simulink model "ElevatorPlant_basic"  (R2015b)
(part 3 of 3)

          Emergency.OpCl.OpCl_1.Closing1.Flag_floor -> (junction 23694)
          (junction 23694) -> (junction 23693)
          (junction 23693) -> (junction 23696)
          Emergency.OpCl.OpCl_1.Closing1.Stop_Closing1 -> (junction 23695)
          (junction 23695) -> (junction 23696)
        state StopClosing
          en: CP1=false;
          FLAG_OD=false;
        state Opening1
          state Opening
            en:AP1=Q_op;
          state Stop_Opening
            en:AP1=false;
            FLAG_OD=true;
            OBS=true;
            IN_op=false;
            ET_op=0;
          state Timer_open
            state Set_tmr
              en: Q_op=true;
            state Set
              en:PT_op=2;
              IN_op=true;
            state Counting
              en:ET_op = ET_op + 1;
              Q_op=false;
            (junction 23815) -> Emergency.OpCl.OpCl_1.Opening1.Timer_open.Set_tmr [order 1] : [ET_op==PT_op]
            Emergency.OpCl.OpCl_1.Opening1.Timer_open.Set_tmr -> (junction 23816)
            (default) -> Emergency.OpCl.OpCl_1.Opening1.Timer_open.Set
            Emergency.OpCl.OpCl_1.Opening1.Timer_open.Counting -> (junction 23815)
            (junction 23815) -> (junction 23816) [order 2]
            Emergency.OpCl.OpCl_1.Opening1.Timer_open.Set -> (junction 23817)
            (junction 23817) -> Emergency.OpCl.OpCl_1.Opening1.Timer_open.Counting [order 1] : [ET_op<PT_op]
            (junction 23817) -> (junction 23816) [order 2]
          state BUTT_Temp
            state Butt_temp0
              en: BUT_TEMP = 0;
              FLAG_BT=true;
              LPC0=true;
            state Butt_temp1
              en: BUT_TEMP = 1;
              FLAG_BT=true;
              LPC1=true;
            state Butt_temp2
              en: BUT_TEMP = 2;
              FLAG_BT=true;
              LPC2=true;
            state Butt_temp3
              en: BUT_TEMP = 3;
              FLAG_BT=true;
              LPC3=true;
            (default) -> (junction 23830)
            (junction 23830) -> (junction 23831) [order 1] : [not(FLAG_BT)]
            (junction 23831) -> Emergency.OpCl.OpCl_1.Opening1.BUTT_Temp.Butt_temp0 [order 1] : [P0]
            Emergency.OpCl.OpCl_1.Opening1.BUTT_Temp.Butt_temp0 -> (junction 23832)
            (junction 23831) -> (junction 23834) [order 2]
            (junction 23832) -> (junction 23833)
            (junction 23830) -> (junction 23841) [order 2]
            Emergency.OpCl.OpCl_1.Opening1.BUTT_Temp.Butt_temp1 -> (junction 23833)
            (junction 23834) -> Emergency.OpCl.OpCl_1.Opening1.BUTT_Temp.Butt_temp1 [order 1] : [P1]
            (junction 23833) -> (junction 23836)
            (junction 23834) -> (junction 23835) [order 2]
            (junction 23835) -> Emergency.OpCl.OpCl_1.Opening1.BUTT_Temp.Butt_temp2 [order 1] : [P2]
            Emergency.OpCl.OpCl_1.Opening1.BUTT_Temp.Butt_temp2 -> (junction 23836)
            (junction 23835) -> (junction 23837) [order 2]
            (junction 23836) -> (junction 23838)
            (junction 23837) -> Emergency.OpCl.OpCl_1.Opening1.BUTT_Temp.Butt_temp3 [order 1] : [P3]
            Emergency.OpCl.OpCl_1.Opening1.BUTT_Temp.Butt_temp3 -> (junction 23838)
            (junction 23838) -> (junction 23840)
            (junction 23837) -> (junction 23839) [order 2]
            (junction 23840) -> (junction 23839)
            (junction 23839) -> (junction 23842)
            (junction 23841) -> (junction 23842)
          state BUTT_Temp1
            state Butt_temp0
              en: BUT_TEMP = 0;
              FLAG_BT=true;
              LPC0=true;
            state Butt_temp1
              en: BUT_TEMP = 1;
              FLAG_BT=true;
              LPC1=true;
            state Butt_temp2
              en: BUT_TEMP = 2;
              FLAG_BT=true;
              LPC2=true;
            state Butt_temp3
              en: BUT_TEMP = 3;
              FLAG_BT=true;
              LPC3=true;
            (default) -> (junction 23870)
            (junction 23870) -> (junction 23871) [order 1] : [not(FLAG_BT)]
            (junction 23871) -> Emergency.OpCl.OpCl_1.Opening1.BUTT_Temp1.Butt_temp0 [order 1] : [P0]
            Emergency.OpCl.OpCl_1.Opening1.BUTT_Temp1.Butt_temp0 -> (junction 23872)
            (junction 23871) -> (junction 23874) [order 2]
            (junction 23872) -> (junction 23873)
            (junction 23870) -> (junction 23881) [order 2]
            Emergency.OpCl.OpCl_1.Opening1.BUTT_Temp1.Butt_temp1 -> (junction 23873)
            (junction 23874) -> Emergency.OpCl.OpCl_1.Opening1.BUTT_Temp1.Butt_temp1 [order 1] : [P1]
            (junction 23873) -> (junction 23876)
            (junction 23874) -> (junction 23875) [order 2]
            (junction 23875) -> Emergency.OpCl.OpCl_1.Opening1.BUTT_Temp1.Butt_temp2 [order 1] : [P2]
            Emergency.OpCl.OpCl_1.Opening1.BUTT_Temp1.Butt_temp2 -> (junction 23876)
            (junction 23875) -> (junction 23877) [order 2]
            (junction 23876) -> (junction 23878)
            (junction 23877) -> Emergency.OpCl.OpCl_1.Opening1.BUTT_Temp1.Butt_temp3 [order 1] : [P3]
            Emergency.OpCl.OpCl_1.Opening1.BUTT_Temp1.Butt_temp3 -> (junction 23878)
            (junction 23878) -> (junction 23880)
            (junction 23877) -> (junction 23879) [order 2]
            (junction 23880) -> (junction 23879)
            (junction 23879) -> (junction 23882)
            (junction 23881) -> (junction 23882)
          state Opening1
            en:AP1=true;
          state People_IN
            state Check_People_IN
              en:
              COUNTER_IN=false;
            state Ready_IN
              en:
              IN_DEL_IN=false;
              ET_DEL_IN=0;
            state People_KID_IN
              en:
              WEIGHT=WEIGHT+30;
              KIDS=KIDS+1;
            state DELAY_IN
              state Set_tmr
                en:
                Q_DEL_IN=true;
              state Counting
                en:
                ET_DEL_IN = ET_DEL_IN + 1;
                Q_DEL_IN=false;
              state Set
                en:
                IN_DEL_IN=true;
                PT_DEL_IN=0.05;
              (junction 23966) -> Emergency.OpCl.OpCl_1.Opening1.People_IN.DELAY_IN.Set_tmr [order 1] : [ET_DEL_IN==PT_DEL_IN]
              Emergency.OpCl.OpCl_1.Opening1.People_IN.DELAY_IN.Set_tmr -> (junction 23967)
              Emergency.OpCl.OpCl_1.Opening1.People_IN.DELAY_IN.Counting -> (junction 23966)
              (junction 23966) -> (junction 23967) [order 2]
              (default) -> Emergency.OpCl.OpCl_1.Opening1.People_IN.DELAY_IN.Set
              Emergency.OpCl.OpCl_1.Opening1.People_IN.DELAY_IN.Set -> (junction 23968)
              (junction 23968) -> Emergency.OpCl.OpCl_1.Opening1.People_IN.DELAY_IN.Counting [order 1] : [ET_DEL_IN<PT_DEL_IN]
              (junction 23968) -> (junction 23967) [order 2]
            state People_WOMAN_IN
              en:
              WEIGHT=WEIGHT+55;
              WOMEN=WOMEN+1;
            state People_MAN_IN
              en:
              WEIGHT=WEIGHT+75;
              MEN=MEN+1;
            state People_FATGUY_IN
              en:
              WEIGHT=WEIGHT+100;
              FATGUYS=FATGUYS+1;
            state Re_Ready_IN
              en:
              COUNTER_IN=true;
            Emergency.OpCl.OpCl_1.Opening1.People_IN.Check_People_IN -> (junction 23911)
            (junction 23911) -> Emergency.OpCl.OpCl_1.Opening1.People_IN.People_KID_IN [order 1] : [KID_IN]
            Emergency.OpCl.OpCl_1.Opening1.People_IN.People_KID_IN -> (junction 23912)
            Emergency.OpCl.OpCl_1.Opening1.People_IN.DELAY_IN -> (junction 23913)
            (junction 23913) -> Emergency.OpCl.OpCl_1.Opening1.People_IN.Ready_IN [order 1] : [Q_DEL_IN]
            (default) -> Emergency.OpCl.OpCl_1.Opening1.People_IN.DELAY_IN
            Emergency.OpCl.OpCl_1.Opening1.People_IN.Ready_IN -> (junction 23914)
            (junction 23914) -> Emergency.OpCl.OpCl_1.Opening1.People_IN.Check_People_IN [order 1] : [COUNTER_IN]
            (junction 23911) -> (junction 23916) [order 2]
            (junction 23912) -> (junction 23915)
            (junction 23913) -> (junction 23925) [order 2]
            (junction 23914) -> (junction 23924) [order 2]
            (junction 23916) -> Emergency.OpCl.OpCl_1.Opening1.People_IN.People_WOMAN_IN [order 1] : [WOMAN_IN]
            Emergency.OpCl.OpCl_1.Opening1.People_IN.People_WOMAN_IN -> (junction 23915)
            (junction 23916) -> (junction 23917) [order 2]
            (junction 23915) -> (junction 23918)
            (junction 23917) -> Emergency.OpCl.OpCl_1.Opening1.People_IN.People_MAN_IN [order 1] : [MAN_IN]
            Emergency.OpCl.OpCl_1.Opening1.People_IN.People_MAN_IN -> (junction 23918)
            (junction 23917) -> (junction 23919) [order 2]
            (junction 23918) -> (junction 23920)
            (junction 23919) -> Emergency.OpCl.OpCl_1.Opening1.People_IN.People_FATGUY_IN [order 1] : [FATGUY_IN]
            Emergency.OpCl.OpCl_1.Opening1.People_IN.People_FATGUY_IN -> (junction 23920)
            (junction 23919) -> (junction 23921) [order 2]
            (junction 23920) -> (junction 23922)
            (junction 23921) -> (junction 23922)
            (junction 23922) -> (junction 23923)
            (junction 23924) -> (junction 23923)
            (junction 23923) -> (junction 23926)
            (junction 23925) -> (junction 23926)
            (junction 23926) -> (junction 23927)
            (junction 23927) -> Emergency.OpCl.OpCl_1.Opening1.People_IN.Re_Ready_IN [order 1] : [not(KID_IN|| WOMAN_IN || MAN_IN || FATGUY_IN)]
            (junction 23927) -> (junction 23928) [order 2]
            Emergency.OpCl.OpCl_1.Opening1.People_IN.Re_Ready_IN -> (junction 23928)
          state People_OUT
            state Ready_OUT
              en:
              IN_DEL_OUT=false;
              ET_DEL_OUT=0;
            state Check_People_OUT
              en:
              COUNTER_OUT=false;
            state People_KID_OUT
              en:
              WEIGHT=WEIGHT-30;
              KIDS=KIDS-1;
            state DELAY_OUT
              state Set_tmr
                en:
                Q_DEL_OUT=true;
              state Counting
                en:
                ET_DEL_OUT = ET_DEL_OUT + 1;
                Q_DEL_OUT=false;
              state Set
                en:
                IN_DEL_OUT=true;
                PT_DEL_OUT=0.05;
              (junction 24040) -> Emergency.OpCl.OpCl_1.Opening1.People_OUT.DELAY_OUT.Set_tmr [order 1] : [ET_DEL_OUT==PT_DEL_OUT]
              Emergency.OpCl.OpCl_1.Opening1.People_OUT.DELAY_OUT.Set_tmr -> (junction 24041)
              Emergency.OpCl.OpCl_1.Opening1.People_OUT.DELAY_OUT.Counting -> (junction 24040)
              (junction 24040) -> (junction 24041) [order 2]
              (default) -> Emergency.OpCl.OpCl_1.Opening1.People_OUT.DELAY_OUT.Set
              Emergency.OpCl.OpCl_1.Opening1.People_OUT.DELAY_OUT.Set -> (junction 24042)
              (junction 24042) -> Emergency.OpCl.OpCl_1.Opening1.People_OUT.DELAY_OUT.Counting [order 1] : [ET_DEL_OUT<PT_DEL_OUT]
              (junction 24042) -> (junction 24041) [order 2]
            state People_WOMAN_OUT
              en:
              WEIGHT=WEIGHT-55;
              WOMEN=WOMEN-1;
            state People_MAN_OUT
              en:
              WEIGHT=WEIGHT-75;
              MEN=MEN-1;
            state People_FATGUY_OUT
              en:
              WEIGHT=WEIGHT-100;
              FATGUYS=FATGUYS-1;
            state Re_Ready_OUT
              en:
              COUNTER_OUT=true;
            (default) -> Emergency.OpCl.OpCl_1.Opening1.People_OUT.DELAY_OUT
            Emergency.OpCl.OpCl_1.Opening1.People_OUT.DELAY_OUT -> (junction 23985)
            (junction 23985) -> Emergency.OpCl.OpCl_1.Opening1.People_OUT.Ready_OUT [order 1] : [Q_DEL_OUT]
            Emergency.OpCl.OpCl_1.Opening1.People_OUT.Ready_OUT -> (junction 23986)
            (junction 23986) -> Emergency.OpCl.OpCl_1.Opening1.People_OUT.Check_People_OUT [order 1] : [COUNTER_OUT]
            Emergency.OpCl.OpCl_1.Opening1.People_OUT.Check_People_OUT -> (junction 23987)
            (junction 23987) -> Emergency.OpCl.OpCl_1.Opening1.People_OUT.People_KID_OUT [order 1] : [KID_OUT && KIDS>0 ]
            Emergency.OpCl.OpCl_1.Opening1.People_OUT.People_KID_OUT -> (junction 23988)
            (junction 23985) -> (junction 23999) [order 2]
            (junction 23986) -> (junction 23997) [order 2]
            (junction 23987) -> (junction 23989) [order 2]
            (junction 23988) -> (junction 23990)
            (junction 23989) -> Emergency.OpCl.OpCl_1.Opening1.People_OUT.People_WOMAN_OUT [order 1] : [WOMAN_OUT && WOMEN>0]
            Emergency.OpCl.OpCl_1.Opening1.People_OUT.People_WOMAN_OUT -> (junction 23990)
            (junction 23989) -> (junction 23992) [order 2]
            (junction 23990) -> (junction 23991)
            (junction 23992) -> Emergency.OpCl.OpCl_1.Opening1.People_OUT.People_MAN_OUT [order 1] : [MAN_OUT && MEN>0]
            Emergency.OpCl.OpCl_1.Opening1.People_OUT.People_MAN_OUT -> (junction 23991)
            (junction 23992) -> (junction 23993) [order 2]
            (junction 23991) -> (junction 23994)
            (junction 23993) -> Emergency.OpCl.OpCl_1.Opening1.People_OUT.People_FATGUY_OUT [order 1] : [FATGUY_OUT && FATGUYS>0]
            Emergency.OpCl.OpCl_1.Opening1.People_OUT.People_FATGUY_OUT -> (junction 23994)
            (junction 23993) -> (junction 23996) [order 2]
            (junction 23994) -> (junction 23995)
            (junction 23996) -> (junction 23995)
            (junction 23995) -> (junction 23998)
            (junction 23997) -> (junction 23998)
            (junction 23998) -> (junction 24000)
            (junction 23999) -> (junction 24000)
            (junction 24000) -> (junction 24001)
            (junction 24001) -> Emergency.OpCl.OpCl_1.Opening1.People_OUT.Re_Ready_OUT [order 1] : [not(KID_OUT || WOMAN_OUT || MAN_OUT || FATGUY_OUT)]
            (junction 24001) -> (junction 24002) [order 2]
            Emergency.OpCl.OpCl_1.Opening1.People_OUT.Re_Ready_OUT -> (junction 24002)
          state Stop_Opening1
            en: AP1=false;
            FLAG_OD=true;
            IN_cl=false;
            ET_cl=0;
          Emergency.OpCl.OpCl_1.Opening1.Opening -> (junction 23781)
          (junction 23781) -> (junction 23780)
          Emergency.OpCl.OpCl_1.Opening1.Stop_Opening -> (junction 23781)
          (junction 23780) -> (junction 23784)
          (junction 23783) -> Emergency.OpCl.OpCl_1.Opening1.Opening [order 1] : [not(PA1)]
          (junction 23782) -> Emergency.OpCl.OpCl_1.Opening1.BUTT_Temp [order 1] : [not(FLAG==4)]
          Emergency.OpCl.OpCl_1.Opening1.BUTT_Temp -> (junction 23783)
          (junction 23783) -> Emergency.OpCl.OpCl_1.Opening1.Stop_Opening [order 2]
          Emergency.OpCl.OpCl_1.Opening1.Timer_open -> (junction 23782)
          (junction 23782) -> (junction 23783) [order 2]
          (junction 23786) -> Emergency.OpCl.OpCl_1.Opening1.Timer_open [order 1] : [not(OBS)]
          Emergency.OpCl.OpCl_1.Opening1.Opening1 -> (junction 23784)
          (junction 23785) -> Emergency.OpCl.OpCl_1.Opening1.Opening1 [order 1] : [not(PA1)]
          Emergency.OpCl.OpCl_1.Opening1.BUTT_Temp1 -> (junction 23785)
          Emergency.OpCl.OpCl_1.Opening1.People_IN -> Emergency.OpCl.OpCl_1.Opening1.People_OUT
          Emergency.OpCl.OpCl_1.Opening1.People_OUT -> (junction 23786)
          (junction 23786) -> (junction 23787) [order 2]
          (junction 23787) -> Emergency.OpCl.OpCl_1.Opening1.BUTT_Temp1 [order 1] : [not(FLAG==4)]
          (default) -> Emergency.OpCl.OpCl_1.Opening1.People_IN
          (junction 23787) -> (junction 23785) [order 2]
          (junction 23788) -> (junction 23784)
          (junction 23785) -> Emergency.OpCl.OpCl_1.Opening1.Stop_Opening1 [order 2]
          Emergency.OpCl.OpCl_1.Opening1.Stop_Opening1 -> (junction 23788)
        (default) -> (junction 23673)
        (junction 23673) -> (junction 23674) [order 1] : [FLAG_OD]
        (junction 23674) -> Emergency.OpCl.OpCl_1.Closing1 [order 1] : [not(SWITCH) && not(STOP) && WEIGHT<=320 && not(PS1 || PD1 || P1) ]
        (junction 23673) -> Emergency.OpCl.OpCl_1.Opening1 [order 2]
        (junction 23674) -> Emergency.OpCl.OpCl_1.StopClosing [order 2]
        Emergency.OpCl.OpCl_1.Closing1 -> (junction 23675)
        Emergency.OpCl.OpCl_1.StopClosing -> (junction 23675)
        (junction 23675) -> (junction 23676)
        Emergency.OpCl.OpCl_1.Opening1 -> (junction 23676)
      state FLOOR_2
        en: CP2=false;
      state OpCl_2
        state Closing2
          state Timer_close
            state Set_tmr
              en: Q_cl=true;
            state Set
              en:PT_cl=5;
              IN_cl=true;
            state Counting
              en:ET_cl = ET_cl + 1;
              Q_cl=false;
            (junction 24494) -> Emergency.OpCl.OpCl_2.Closing2.Timer_close.Set_tmr [order 1] : [ET_cl==PT_cl]
            Emergency.OpCl.OpCl_2.Closing2.Timer_close.Set_tmr -> (junction 24495)
            (default) -> Emergency.OpCl.OpCl_2.Closing2.Timer_close.Set
            Emergency.OpCl.OpCl_2.Closing2.Timer_close.Counting -> (junction 24494)
            (junction 24494) -> (junction 24495) [order 2]
            Emergency.OpCl.OpCl_2.Closing2.Timer_close.Set -> (junction 24496)
            (junction 24496) -> Emergency.OpCl.OpCl_2.Closing2.Timer_close.Counting [order 1] : [ET_cl<PT_cl]
            (junction 24496) -> (junction 24495) [order 2]
          state BUTT_Temp
            state Butt_temp0
              en: BUT_TEMP = 0;
              FLAG_BT=true;
              LPC0=true;
            state Butt_temp1
              en: BUT_TEMP = 1;
              FLAG_BT=true;
              LPC1=true;
            state Butt_temp2
              en: BUT_TEMP = 2;
              FLAG_BT=true;
              LPC2=true;
            state Butt_temp3
              en: BUT_TEMP = 3;
              FLAG_BT=true;
              LPC3=true;
            (default) -> (junction 24509)
            (junction 24509) -> (junction 24510) [order 1] : [not(FLAG_BT)]
            (junction 24510) -> Emergency.OpCl.OpCl_2.Closing2.BUTT_Temp.Butt_temp0 [order 1] : [P0]
            Emergency.OpCl.OpCl_2.Closing2.BUTT_Temp.Butt_temp0 -> (junction 24511)
            (junction 24509) -> (junction 24518) [order 2]
            (junction 24510) -> (junction 24513) [order 2]
            (junction 24511) -> (junction 24512)
            (junction 24513) -> Emergency.OpCl.OpCl_2.Closing2.BUTT_Temp.Butt_temp1 [order 1] : [P1]
            Emergency.OpCl.OpCl_2.Closing2.BUTT_Temp.Butt_temp1 -> (junction 24512)
            (junction 24513) -> (junction 24514) [order 2]
            (junction 24512) -> (junction 24515)
            (junction 24514) -> Emergency.OpCl.OpCl_2.Closing2.BUTT_Temp.Butt_temp2 [order 1] : [P2]
            Emergency.OpCl.OpCl_2.Closing2.BUTT_Temp.Butt_temp2 -> (junction 24515)
            (junction 24514) -> (junction 24516) [order 2]
            (junction 24515) -> (junction 24517)
            (junction 24516) -> Emergency.OpCl.OpCl_2.Closing2.BUTT_Temp.Butt_temp3 [order 1] : [P3]
            Emergency.OpCl.OpCl_2.Closing2.BUTT_Temp.Butt_temp3 -> (junction 24517)
            (junction 24516) -> (junction 24519) [order 2]
            (junction 24517) -> (junction 24520)
            (junction 24518) -> (junction 24519)
            (junction 24519) -> (junction 24520)
          state Closing
            en: CP2=Q_cl;
          state Stop_Closing
            en: CP2=false;
            LPS0=false;
            LPS1=false;
            LPD1=false;
            LPS2=false;
            LPD2=false;
            LPD3=false;
            FLAG_OD=false;
            OBS=false;
            ET_cl=0;
            IN_cl=false;
          state Flag_position
            en:FLAG=2;
            FLAG_BT=false;
            BUTTON=BUT_TEMP;
          state Closing1
            en:CP2=true;
          state Flag_floor
            en: FLAG=1;
          state Stop_Closing1
            en:CP2=false;
          Emergency.OpCl.OpCl_2.Closing2.Closing -> Emergency.OpCl.OpCl_2.Closing2.BUTT_Temp
          (default) -> (junction 24461)
          (junction 24461) -> Emergency.OpCl.OpCl_2.Closing2.Timer_close [order 1] : [not(FLAG==0) && not(FLAG==4)]
          Emergency.OpCl.OpCl_2.Closing2.Timer_close -> (junction 24462)
          Emergency.OpCl.OpCl_2.Closing2.BUTT_Temp -> (junction 24463)
          (junction 24462) -> Emergency.OpCl.OpCl_2.Closing2.Closing [order 1] : [not(PC2)]
          (junction 24461) -> (junction 24465) [order 2]
          (junction 24462) -> Emergency.OpCl.OpCl_2.Closing2.Stop_Closing [order 2]
          (junction 24463) -> (junction 24467)
          Emergency.OpCl.OpCl_2.Closing2.Stop_Closing -> (junction 24464)
          (junction 24464) -> Emergency.OpCl.OpCl_2.Closing2.Flag_position [order 1] : [FLAG_BT]
          (junction 24464) -> Emergency.OpCl.OpCl_2.Closing2.Flag_floor [order 2]
          Emergency.OpCl.OpCl_2.Closing2.Flag_position -> (junction 24468)
          (junction 24465) -> Emergency.OpCl.OpCl_2.Closing2.Closing1 [order 1] : [not(PC2)]
          Emergency.OpCl.OpCl_2.Closing2.Closing1 -> (junction 24466)
          (junction 24465) -> Emergency.OpCl.OpCl_2.Closing2.Stop_Closing1 [order 2]
          (junction 24466) -> (junction 24469)
          Emergency.OpCl.OpCl_2.Closing2.Flag_floor -> (junction 24468)
          (junction 24468) -> (junction 24467)
          (junction 24467) -> (junction 24470)
          Emergency.OpCl.OpCl_2.Closing2.Stop_Closing1 -> (junction 24469)
          (junction 24469) -> (junction 24470)
        state StopClosing
          en: CP2=false;
          FLAG_OD=false;
        state Opening2
          state Opening
            en:AP2=Q_op;
          state Stop_Opening
            en:AP2=false;
            FLAG_OD=true;
            OBS=true;
            IN_op=false;
            ET_op=0;
          state Timer_open
            state Set_tmr
              en: Q_op=true;
            state Set
              en:PT_op=2;
              IN_op=true;
            state Counting
              en:ET_op = ET_op + 1;
              Q_op=false;
            (junction 24589) -> Emergency.OpCl.OpCl_2.Opening2.Timer_open.Set_tmr [order 1] : [ET_op==PT_op]
            Emergency.OpCl.OpCl_2.Opening2.Timer_open.Set_tmr -> (junction 24590)
            (default) -> Emergency.OpCl.OpCl_2.Opening2.Timer_open.Set
            Emergency.OpCl.OpCl_2.Opening2.Timer_open.Counting -> (junction 24589)
            (junction 24589) -> (junction 24590) [order 2]
            Emergency.OpCl.OpCl_2.Opening2.Timer_open.Set -> (junction 24591)
            (junction 24591) -> Emergency.OpCl.OpCl_2.Opening2.Timer_open.Counting [order 1] : [ET_op<PT_op]
            (junction 24591) -> (junction 24590) [order 2]
          state BUTT_Temp
            state Butt_temp0
              en: BUT_TEMP = 0;
              FLAG_BT=true;
              LPC0=true;
            state Butt_temp1
              en: BUT_TEMP = 1;
              FLAG_BT=true;
              LPC1=true;
            state Butt_temp2
              en: BUT_TEMP = 2;
              FLAG_BT=true;
              LPC2=true;
            state Butt_temp3
              en: BUT_TEMP = 3;
              FLAG_BT=true;
              LPC3=true;
            (default) -> (junction 24604)
            (junction 24604) -> (junction 24605) [order 1] : [not(FLAG_BT)]
            (junction 24605) -> Emergency.OpCl.OpCl_2.Opening2.BUTT_Temp.Butt_temp0 [order 1] : [P0]
            Emergency.OpCl.OpCl_2.Opening2.BUTT_Temp.Butt_temp0 -> (junction 24606)
            (junction 24605) -> (junction 24608) [order 2]
            (junction 24606) -> (junction 24607)
            (junction 24604) -> (junction 24615) [order 2]
            Emergency.OpCl.OpCl_2.Opening2.BUTT_Temp.Butt_temp1 -> (junction 24607)
            (junction 24608) -> Emergency.OpCl.OpCl_2.Opening2.BUTT_Temp.Butt_temp1 [order 1] : [P1]
            (junction 24607) -> (junction 24610)
            (junction 24608) -> (junction 24609) [order 2]
            (junction 24609) -> Emergency.OpCl.OpCl_2.Opening2.BUTT_Temp.Butt_temp2 [order 1] : [P2]
            Emergency.OpCl.OpCl_2.Opening2.BUTT_Temp.Butt_temp2 -> (junction 24610)
            (junction 24609) -> (junction 24611) [order 2]
            (junction 24610) -> (junction 24612)
            (junction 24611) -> Emergency.OpCl.OpCl_2.Opening2.BUTT_Temp.Butt_temp3 [order 1] : [P3]
            Emergency.OpCl.OpCl_2.Opening2.BUTT_Temp.Butt_temp3 -> (junction 24612)
            (junction 24612) -> (junction 24614)
            (junction 24611) -> (junction 24613) [order 2]
            (junction 24614) -> (junction 24613)
            (junction 24613) -> (junction 24616)
            (junction 24615) -> (junction 24616)
          state BUTT_Temp1
            state Butt_temp0
              en: BUT_TEMP = 0;
              FLAG_BT=true;
              LPC0=true;
            state Butt_temp1
              en: BUT_TEMP = 1;
              FLAG_BT=true;
              LPC1=true;
            state Butt_temp2
              en: BUT_TEMP = 2;
              FLAG_BT=true;
              LPC2=true;
            state Butt_temp3
              en: BUT_TEMP = 3;
              FLAG_BT=true;
              LPC3=true;
            (default) -> (junction 24644)
            (junction 24644) -> (junction 24645) [order 1] : [not(FLAG_BT)]
            (junction 24645) -> Emergency.OpCl.OpCl_2.Opening2.BUTT_Temp1.Butt_temp0 [order 1] : [P0]
            Emergency.OpCl.OpCl_2.Opening2.BUTT_Temp1.Butt_temp0 -> (junction 24646)
            (junction 24645) -> (junction 24648) [order 2]
            (junction 24646) -> (junction 24647)
            (junction 24644) -> (junction 24655) [order 2]
            Emergency.OpCl.OpCl_2.Opening2.BUTT_Temp1.Butt_temp1 -> (junction 24647)
            (junction 24648) -> Emergency.OpCl.OpCl_2.Opening2.BUTT_Temp1.Butt_temp1 [order 1] : [P1]
            (junction 24647) -> (junction 24650)
            (junction 24648) -> (junction 24649) [order 2]
            (junction 24649) -> Emergency.OpCl.OpCl_2.Opening2.BUTT_Temp1.Butt_temp2 [order 1] : [P2]
            Emergency.OpCl.OpCl_2.Opening2.BUTT_Temp1.Butt_temp2 -> (junction 24650)
            (junction 24649) -> (junction 24651) [order 2]
            (junction 24650) -> (junction 24652)
            (junction 24651) -> Emergency.OpCl.OpCl_2.Opening2.BUTT_Temp1.Butt_temp3 [order 1] : [P3]
            Emergency.OpCl.OpCl_2.Opening2.BUTT_Temp1.Butt_temp3 -> (junction 24652)
            (junction 24652) -> (junction 24654)
            (junction 24651) -> (junction 24653) [order 2]
            (junction 24654) -> (junction 24653)
            (junction 24653) -> (junction 24656)
            (junction 24655) -> (junction 24656)
          state Opening1
            en:AP2=true;
          state People_IN
            state Check_People_IN
              en:
              COUNTER_IN=false;
            state Ready_IN
              en:
              IN_DEL_IN=false;
              ET_DEL_IN=0;
            state People_KID_IN
              en:
              WEIGHT=WEIGHT+30;
              KIDS=KIDS+1;
            state DELAY_IN
              state Set_tmr
                en:
                Q_DEL_IN=true;
              state Counting
                en:
                ET_DEL_IN = ET_DEL_IN + 1;
                Q_DEL_IN=false;
              state Set
                en:
                IN_DEL_IN=true;
                PT_DEL_IN=0.05;
              (junction 24740) -> Emergency.OpCl.OpCl_2.Opening2.People_IN.DELAY_IN.Set_tmr [order 1] : [ET_DEL_IN==PT_DEL_IN]
              Emergency.OpCl.OpCl_2.Opening2.People_IN.DELAY_IN.Set_tmr -> (junction 24741)
              Emergency.OpCl.OpCl_2.Opening2.People_IN.DELAY_IN.Counting -> (junction 24740)
              (junction 24740) -> (junction 24741) [order 2]
              (default) -> Emergency.OpCl.OpCl_2.Opening2.People_IN.DELAY_IN.Set
              Emergency.OpCl.OpCl_2.Opening2.People_IN.DELAY_IN.Set -> (junction 24742)
              (junction 24742) -> Emergency.OpCl.OpCl_2.Opening2.People_IN.DELAY_IN.Counting [order 1] : [ET_DEL_IN<PT_DEL_IN]
              (junction 24742) -> (junction 24741) [order 2]
            state People_WOMAN_IN
              en:
              WEIGHT=WEIGHT+55;
              WOMEN=WOMEN+1;
            state People_MAN_IN
              en:
              WEIGHT=WEIGHT+75;
              MEN=MEN+1;
            state People_FATGUY_IN
              en:
              WEIGHT=WEIGHT+100;
              FATGUYS=FATGUYS+1;
            state Re_Ready_IN
              en:
              COUNTER_IN=true;
            Emergency.OpCl.OpCl_2.Opening2.People_IN.Check_People_IN -> (junction 24685)
            (junction 24685) -> Emergency.OpCl.OpCl_2.Opening2.People_IN.People_KID_IN [order 1] : [KID_IN]
            Emergency.OpCl.OpCl_2.Opening2.People_IN.People_KID_IN -> (junction 24686)
            Emergency.OpCl.OpCl_2.Opening2.People_IN.DELAY_IN -> (junction 24687)
            (junction 24687) -> Emergency.OpCl.OpCl_2.Opening2.People_IN.Ready_IN [order 1] : [Q_DEL_IN]
            (default) -> Emergency.OpCl.OpCl_2.Opening2.People_IN.DELAY_IN
            Emergency.OpCl.OpCl_2.Opening2.People_IN.Ready_IN -> (junction 24688)
            (junction 24688) -> Emergency.OpCl.OpCl_2.Opening2.People_IN.Check_People_IN [order 1] : [COUNTER_IN]
            (junction 24685) -> (junction 24690) [order 2]
            (junction 24686) -> (junction 24689)
            (junction 24687) -> (junction 24699) [order 2]
            (junction 24688) -> (junction 24698) [order 2]
            (junction 24690) -> Emergency.OpCl.OpCl_2.Opening2.People_IN.People_WOMAN_IN [order 1] : [WOMAN_IN]
            Emergency.OpCl.OpCl_2.Opening2.People_IN.People_WOMAN_IN -> (junction 24689)
            (junction 24690) -> (junction 24691) [order 2]
            (junction 24689) -> (junction 24692)
            (junction 24691) -> Emergency.OpCl.OpCl_2.Opening2.People_IN.People_MAN_IN [order 1] : [MAN_IN]
            Emergency.OpCl.OpCl_2.Opening2.People_IN.People_MAN_IN -> (junction 24692)
            (junction 24691) -> (junction 24693) [order 2]
            (junction 24692) -> (junction 24694)
            (junction 24693) -> Emergency.OpCl.OpCl_2.Opening2.People_IN.People_FATGUY_IN [order 1] : [FATGUY_IN]
            Emergency.OpCl.OpCl_2.Opening2.People_IN.People_FATGUY_IN -> (junction 24694)
            (junction 24693) -> (junction 24695) [order 2]
            (junction 24694) -> (junction 24696)
            (junction 24695) -> (junction 24696)
            (junction 24696) -> (junction 24697)
            (junction 24698) -> (junction 24697)
            (junction 24697) -> (junction 24700)
            (junction 24699) -> (junction 24700)
            (junction 24700) -> (junction 24701)
            (junction 24701) -> Emergency.OpCl.OpCl_2.Opening2.People_IN.Re_Ready_IN [order 1] : [not(KID_IN|| WOMAN_IN || MAN_IN || FATGUY_IN)]
            (junction 24701) -> (junction 24702) [order 2]
            Emergency.OpCl.OpCl_2.Opening2.People_IN.Re_Ready_IN -> (junction 24702)
          state People_OUT
            state Ready_OUT
              en:
              IN_DEL_OUT=false;
              ET_DEL_OUT=0;
            state Check_People_OUT
              en:
              COUNTER_OUT=false;
            state People_KID_OUT
              en:
              WEIGHT=WEIGHT-30;
              KIDS=KIDS-1;
            state DELAY_OUT
              state Set_tmr
                en:
                Q_DEL_OUT=true;
              state Counting
                en:
                ET_DEL_OUT = ET_DEL_OUT + 1;
                Q_DEL_OUT=false;
              state Set
                en:
                IN_DEL_OUT=true;
                PT_DEL_OUT=0.05;
              (junction 24814) -> Emergency.OpCl.OpCl_2.Opening2.People_OUT.DELAY_OUT.Set_tmr [order 1] : [ET_DEL_OUT==PT_DEL_OUT]
              Emergency.OpCl.OpCl_2.Opening2.People_OUT.DELAY_OUT.Set_tmr -> (junction 24815)
              Emergency.OpCl.OpCl_2.Opening2.People_OUT.DELAY_OUT.Counting -> (junction 24814)
              (junction 24814) -> (junction 24815) [order 2]
              (default) -> Emergency.OpCl.OpCl_2.Opening2.People_OUT.DELAY_OUT.Set
              Emergency.OpCl.OpCl_2.Opening2.People_OUT.DELAY_OUT.Set -> (junction 24816)
              (junction 24816) -> Emergency.OpCl.OpCl_2.Opening2.People_OUT.DELAY_OUT.Counting [order 1] : [ET_DEL_OUT<PT_DEL_OUT]
              (junction 24816) -> (junction 24815) [order 2]
            state People_WOMAN_OUT
              en:
              WEIGHT=WEIGHT-55;
              WOMEN=WOMEN-1;
            state People_MAN_OUT
              en:
              WEIGHT=WEIGHT-75;
              MEN=MEN-1;
            state People_FATGUY_OUT
              en:
              WEIGHT=WEIGHT-100;
              FATGUYS=FATGUYS-1;
            state Re_Ready_OUT
              en:
              COUNTER_OUT=true;
            (default) -> Emergency.OpCl.OpCl_2.Opening2.People_OUT.DELAY_OUT
            Emergency.OpCl.OpCl_2.Opening2.People_OUT.DELAY_OUT -> (junction 24759)
            (junction 24759) -> Emergency.OpCl.OpCl_2.Opening2.People_OUT.Ready_OUT [order 1] : [Q_DEL_OUT]
            Emergency.OpCl.OpCl_2.Opening2.People_OUT.Ready_OUT -> (junction 24760)
            (junction 24760) -> Emergency.OpCl.OpCl_2.Opening2.People_OUT.Check_People_OUT [order 1] : [COUNTER_OUT]
            Emergency.OpCl.OpCl_2.Opening2.People_OUT.Check_People_OUT -> (junction 24761)
            (junction 24761) -> Emergency.OpCl.OpCl_2.Opening2.People_OUT.People_KID_OUT [order 1] : [KID_OUT && KIDS>0 ]
            Emergency.OpCl.OpCl_2.Opening2.People_OUT.People_KID_OUT -> (junction 24762)
            (junction 24759) -> (junction 24773) [order 2]
            (junction 24760) -> (junction 24771) [order 2]
            (junction 24761) -> (junction 24763) [order 2]
            (junction 24762) -> (junction 24764)
            (junction 24763) -> Emergency.OpCl.OpCl_2.Opening2.People_OUT.People_WOMAN_OUT [order 1] : [WOMAN_OUT && WOMEN>0]
            Emergency.OpCl.OpCl_2.Opening2.People_OUT.People_WOMAN_OUT -> (junction 24764)
            (junction 24763) -> (junction 24766) [order 2]
            (junction 24764) -> (junction 24765)
            (junction 24766) -> Emergency.OpCl.OpCl_2.Opening2.People_OUT.People_MAN_OUT [order 1] : [MAN_OUT && MEN>0]
            Emergency.OpCl.OpCl_2.Opening2.People_OUT.People_MAN_OUT -> (junction 24765)
            (junction 24766) -> (junction 24767) [order 2]
            (junction 24765) -> (junction 24768)
            (junction 24767) -> Emergency.OpCl.OpCl_2.Opening2.People_OUT.People_FATGUY_OUT [order 1] : [FATGUY_OUT && FATGUYS>0]
            Emergency.OpCl.OpCl_2.Opening2.People_OUT.People_FATGUY_OUT -> (junction 24768)
            (junction 24767) -> (junction 24770) [order 2]
            (junction 24768) -> (junction 24769)
            (junction 24770) -> (junction 24769)
            (junction 24769) -> (junction 24772)
            (junction 24771) -> (junction 24772)
            (junction 24772) -> (junction 24774)
            (junction 24773) -> (junction 24774)
            (junction 24774) -> (junction 24775)
            (junction 24775) -> Emergency.OpCl.OpCl_2.Opening2.People_OUT.Re_Ready_OUT [order 1] : [not(KID_OUT || WOMAN_OUT || MAN_OUT || FATGUY_OUT)]
            (junction 24775) -> (junction 24776) [order 2]
            Emergency.OpCl.OpCl_2.Opening2.People_OUT.Re_Ready_OUT -> (junction 24776)
          state Stop_Opening1
            en: AP2=false;
            FLAG_OD=true;
            IN_cl=false;
            ET_cl=0;
          Emergency.OpCl.OpCl_2.Opening2.Opening -> (junction 24555)
          (junction 24555) -> (junction 24554)
          Emergency.OpCl.OpCl_2.Opening2.Stop_Opening -> (junction 24555)
          (junction 24554) -> (junction 24558)
          (junction 24557) -> Emergency.OpCl.OpCl_2.Opening2.Opening [order 1] : [not(PA2)]
          Emergency.OpCl.OpCl_2.Opening2.BUTT_Temp -> (junction 24557)
          (junction 24557) -> Emergency.OpCl.OpCl_2.Opening2.Stop_Opening [order 2]
          Emergency.OpCl.OpCl_2.Opening2.Timer_open -> (junction 24556)
          (junction 24556) -> Emergency.OpCl.OpCl_2.Opening2.BUTT_Temp [order 1] : [not(FLAG==4)]
          (junction 24556) -> (junction 24557) [order 2]
          (junction 24560) -> Emergency.OpCl.OpCl_2.Opening2.Timer_open [order 1] : [not(OBS)]
          Emergency.OpCl.OpCl_2.Opening2.Opening1 -> (junction 24558)
          Emergency.OpCl.OpCl_2.Opening2.BUTT_Temp1 -> (junction 24559)
          (junction 24559) -> Emergency.OpCl.OpCl_2.Opening2.Opening1 [order 1] : [not(PA2)]
          Emergency.OpCl.OpCl_2.Opening2.People_IN -> Emergency.OpCl.OpCl_2.Opening2.People_OUT
          Emergency.OpCl.OpCl_2.Opening2.People_OUT -> (junction 24560)
          (junction 24560) -> (junction 24561) [order 2]
          (junction 24561) -> Emergency.OpCl.OpCl_2.Opening2.BUTT_Temp1 [order 1] : [not(FLAG==4)]
          (default) -> Emergency.OpCl.OpCl_2.Opening2.People_IN
          (junction 24561) -> (junction 24559) [order 2]
          (junction 24562) -> (junction 24558)
          (junction 24559) -> Emergency.OpCl.OpCl_2.Opening2.Stop_Opening1 [order 2]
          Emergency.OpCl.OpCl_2.Opening2.Stop_Opening1 -> (junction 24562)
        (default) -> (junction 24447)
        (junction 24447) -> (junction 24448) [order 1] : [FLAG_OD]
        (junction 24448) -> Emergency.OpCl.OpCl_2.Closing2 [order 1] : [not(SWITCH) && not(STOP) && WEIGHT<=320 && not(PS2 || PD2 || P2) ]
        (junction 24447) -> Emergency.OpCl.OpCl_2.Opening2 [order 2]
        (junction 24448) -> Emergency.OpCl.OpCl_2.StopClosing [order 2]
        Emergency.OpCl.OpCl_2.Closing2 -> (junction 24449)
        Emergency.OpCl.OpCl_2.StopClosing -> (junction 24449)
        (junction 24449) -> (junction 24450)
        Emergency.OpCl.OpCl_2.Opening2 -> (junction 24450)
      state FLOOR_3
        en: CP3=false;
      state OpCl_3
        state Closing3
          state Timer_close
            state Set_tmr
              en: Q_cl=true;
            state Set
              en:PT_cl=5;
              IN_cl=true;
            state Counting
              en:ET_cl = ET_cl + 1;
              Q_cl=false;
            (junction 24881) -> Emergency.OpCl.OpCl_3.Closing3.Timer_close.Set_tmr [order 1] : [ET_cl==PT_cl]
            Emergency.OpCl.OpCl_3.Closing3.Timer_close.Set_tmr -> (junction 24882)
            (default) -> Emergency.OpCl.OpCl_3.Closing3.Timer_close.Set
            Emergency.OpCl.OpCl_3.Closing3.Timer_close.Counting -> (junction 24881)
            (junction 24881) -> (junction 24882) [order 2]
            Emergency.OpCl.OpCl_3.Closing3.Timer_close.Set -> (junction 24883)
            (junction 24883) -> Emergency.OpCl.OpCl_3.Closing3.Timer_close.Counting [order 1] : [ET_cl<PT_cl]
            (junction 24883) -> (junction 24882) [order 2]
          state BUTT_Temp
            state Butt_temp0
              en: BUT_TEMP = 0;
              FLAG_BT=true;
              LPC0=true;
            state Butt_temp1
              en: BUT_TEMP = 1;
              FLAG_BT=true;
              LPC1=true;
            state Butt_temp2
              en: BUT_TEMP = 2;
              FLAG_BT=true;
              LPC2=true;
            state Butt_temp3
              en: BUT_TEMP = 3;
              FLAG_BT=true;
              LPC3=true;
            (default) -> (junction 24896)
            (junction 24896) -> (junction 24897) [order 1] : [not(FLAG_BT)]
            (junction 24897) -> Emergency.OpCl.OpCl_3.Closing3.BUTT_Temp.Butt_temp0 [order 1] : [P0]
            Emergency.OpCl.OpCl_3.Closing3.BUTT_Temp.Butt_temp0 -> (junction 24898)
            (junction 24896) -> (junction 24905) [order 2]
            (junction 24897) -> (junction 24900) [order 2]
            (junction 24898) -> (junction 24899)
            (junction 24900) -> Emergency.OpCl.OpCl_3.Closing3.BUTT_Temp.Butt_temp1 [order 1] : [P1]
            Emergency.OpCl.OpCl_3.Closing3.BUTT_Temp.Butt_temp1 -> (junction 24899)
            (junction 24900) -> (junction 24901) [order 2]
            (junction 24899) -> (junction 24902)
            (junction 24901) -> Emergency.OpCl.OpCl_3.Closing3.BUTT_Temp.Butt_temp2 [order 1] : [P2]
            Emergency.OpCl.OpCl_3.Closing3.BUTT_Temp.Butt_temp2 -> (junction 24902)
            (junction 24901) -> (junction 24903) [order 2]
            (junction 24902) -> (junction 24904)
            (junction 24903) -> Emergency.OpCl.OpCl_3.Closing3.BUTT_Temp.Butt_temp3 [order 1] : [P3]
            Emergency.OpCl.OpCl_3.Closing3.BUTT_Temp.Butt_temp3 -> (junction 24904)
            (junction 24903) -> (junction 24906) [order 2]
            (junction 24904) -> (junction 24907)
            (junction 24905) -> (junction 24906)
            (junction 24906) -> (junction 24907)
          state Closing
            en: CP3=Q_cl;
          state Stop_Closing
            en: CP3=false;
            LPS0=false;
            LPS1=false;
            LPD1=false;
            LPS2=false;
            LPD2=false;
            LPD3=false;
            FLAG_OD=false;
            OBS=false;
            ET_cl=0;
            IN_cl=false;
          state Flag_position
            en:FLAG=2;
            FLAG_BT=false;
            BUTTON=BUT_TEMP;
          state Closing1
            en:CP3=true;
          state Flag_floor
            en: FLAG=1;
          state Stop_Closing1
            en:CP3=false;
          Emergency.OpCl.OpCl_3.Closing3.Closing -> Emergency.OpCl.OpCl_3.Closing3.BUTT_Temp
          (default) -> (junction 24848)
          (junction 24848) -> Emergency.OpCl.OpCl_3.Closing3.Timer_close [order 1] : [not(FLAG==0) && not(FLAG==4)]
          Emergency.OpCl.OpCl_3.Closing3.Timer_close -> (junction 24849)
          Emergency.OpCl.OpCl_3.Closing3.BUTT_Temp -> (junction 24850)
          (junction 24849) -> Emergency.OpCl.OpCl_3.Closing3.Closing [order 1] : [not(PC3)]
          (junction 24848) -> (junction 24852) [order 2]
          (junction 24849) -> Emergency.OpCl.OpCl_3.Closing3.Stop_Closing [order 2]
          (junction 24850) -> (junction 24854)
          Emergency.OpCl.OpCl_3.Closing3.Stop_Closing -> (junction 24851)
          (junction 24851) -> Emergency.OpCl.OpCl_3.Closing3.Flag_position [order 1] : [FLAG_BT]
          (junction 24851) -> Emergency.OpCl.OpCl_3.Closing3.Flag_floor [order 2]
          Emergency.OpCl.OpCl_3.Closing3.Flag_position -> (junction 24855)
          (junction 24852) -> Emergency.OpCl.OpCl_3.Closing3.Closing1 [order 1] : [not(PC3)]
          Emergency.OpCl.OpCl_3.Closing3.Closing1 -> (junction 24853)
          (junction 24852) -> Emergency.OpCl.OpCl_3.Closing3.Stop_Closing1 [order 2]
          (junction 24853) -> (junction 24856)
          Emergency.OpCl.OpCl_3.Closing3.Flag_floor -> (junction 24855)
          (junction 24855) -> (junction 24854)
          (junction 24854) -> (junction 24857)
          Emergency.OpCl.OpCl_3.Closing3.Stop_Closing1 -> (junction 24856)
          (junction 24856) -> (junction 24857)
        state StopClosing
          en: CP3=false;
          FLAG_OD=false;
        state Opening3
          state Opening
            en:AP3=Q_op;
          state Stop_Opening
            en:AP3=false;
            FLAG_OD=true;
            OBS=true;
            IN_op=false;
            ET_op=0;
          state Timer_open
            state Set_tmr
              en: Q_op=true;
            state Set
              en:PT_op=2;
              IN_op=true;
            state Counting
              en:ET_op = ET_op + 1;
              Q_op=false;
            (junction 24976) -> Emergency.OpCl.OpCl_3.Opening3.Timer_open.Set_tmr [order 1] : [ET_op==PT_op]
            Emergency.OpCl.OpCl_3.Opening3.Timer_open.Set_tmr -> (junction 24977)
            (default) -> Emergency.OpCl.OpCl_3.Opening3.Timer_open.Set
            Emergency.OpCl.OpCl_3.Opening3.Timer_open.Counting -> (junction 24976)
            (junction 24976) -> (junction 24977) [order 2]
            Emergency.OpCl.OpCl_3.Opening3.Timer_open.Set -> (junction 24978)
            (junction 24978) -> Emergency.OpCl.OpCl_3.Opening3.Timer_open.Counting [order 1] : [ET_op<PT_op]
            (junction 24978) -> (junction 24977) [order 2]
          state BUTT_Temp
            state Butt_temp0
              en: BUT_TEMP = 0;
              FLAG_BT=true;
              LPC0=true;
            state Butt_temp1
              en: BUT_TEMP = 1;
              FLAG_BT=true;
              LPC1=true;
            state Butt_temp2
              en: BUT_TEMP = 2;
              FLAG_BT=true;
              LPC2=true;
            state Butt_temp3
              en: BUT_TEMP = 3;
              FLAG_BT=true;
              LPC3=true;
            (default) -> (junction 24991)
            (junction 24991) -> (junction 24992) [order 1] : [not(FLAG_BT)]
            (junction 24992) -> Emergency.OpCl.OpCl_3.Opening3.BUTT_Temp.Butt_temp0 [order 1] : [P0]
            Emergency.OpCl.OpCl_3.Opening3.BUTT_Temp.Butt_temp0 -> (junction 24993)
            (junction 24992) -> (junction 24995) [order 2]
            (junction 24993) -> (junction 24994)
            (junction 24991) -> (junction 25002) [order 2]
            Emergency.OpCl.OpCl_3.Opening3.BUTT_Temp.Butt_temp1 -> (junction 24994)
            (junction 24995) -> Emergency.OpCl.OpCl_3.Opening3.BUTT_Temp.Butt_temp1 [order 1] : [P1]
            (junction 24994) -> (junction 24997)
            (junction 24995) -> (junction 24996) [order 2]
            (junction 24996) -> Emergency.OpCl.OpCl_3.Opening3.BUTT_Temp.Butt_temp2 [order 1] : [P2]
            Emergency.OpCl.OpCl_3.Opening3.BUTT_Temp.Butt_temp2 -> (junction 24997)
            (junction 24996) -> (junction 24998) [order 2]
            (junction 24997) -> (junction 24999)
            (junction 24998) -> Emergency.OpCl.OpCl_3.Opening3.BUTT_Temp.Butt_temp3 [order 1] : [P3]
            Emergency.OpCl.OpCl_3.Opening3.BUTT_Temp.Butt_temp3 -> (junction 24999)
            (junction 24999) -> (junction 25001)
            (junction 24998) -> (junction 25000) [order 2]
            (junction 25001) -> (junction 25000)
            (junction 25000) -> (junction 25003)
            (junction 25002) -> (junction 25003)
          state BUTT_Temp1
            state Butt_temp0
              en: BUT_TEMP = 0;
              FLAG_BT=true;
              LPC0=true;
            state Butt_temp1
              en: BUT_TEMP = 1;
              FLAG_BT=true;
              LPC1=true;
            state Butt_temp2
              en: BUT_TEMP = 2;
              FLAG_BT=true;
              LPC2=true;
            state Butt_temp3
              en: BUT_TEMP = 3;
              FLAG_BT=true;
              LPC3=true;
            (default) -> (junction 25031)
            (junction 25031) -> (junction 25032) [order 1] : [not(FLAG_BT)]
            (junction 25032) -> Emergency.OpCl.OpCl_3.Opening3.BUTT_Temp1.Butt_temp0 [order 1] : [P0]
            Emergency.OpCl.OpCl_3.Opening3.BUTT_Temp1.Butt_temp0 -> (junction 25033)
            (junction 25032) -> (junction 25035) [order 2]
            (junction 25033) -> (junction 25034)
            (junction 25031) -> (junction 25042) [order 2]
            Emergency.OpCl.OpCl_3.Opening3.BUTT_Temp1.Butt_temp1 -> (junction 25034)
            (junction 25035) -> Emergency.OpCl.OpCl_3.Opening3.BUTT_Temp1.Butt_temp1 [order 1] : [P1]
            (junction 25034) -> (junction 25037)
            (junction 25035) -> (junction 25036) [order 2]
            (junction 25036) -> Emergency.OpCl.OpCl_3.Opening3.BUTT_Temp1.Butt_temp2 [order 1] : [P2]
            Emergency.OpCl.OpCl_3.Opening3.BUTT_Temp1.Butt_temp2 -> (junction 25037)
            (junction 25036) -> (junction 25038) [order 2]
            (junction 25037) -> (junction 25039)
            (junction 25038) -> Emergency.OpCl.OpCl_3.Opening3.BUTT_Temp1.Butt_temp3 [order 1] : [P3]
            Emergency.OpCl.OpCl_3.Opening3.BUTT_Temp1.Butt_temp3 -> (junction 25039)
            (junction 25039) -> (junction 25041)
            (junction 25038) -> (junction 25040) [order 2]
            (junction 25041) -> (junction 25040)
            (junction 25040) -> (junction 25043)
            (junction 25042) -> (junction 25043)
          state Opening1
            en:AP3=true;
          state People_IN
            state Check_People_IN
              en:
              COUNTER_IN=false;
            state Ready_IN
              en:
              IN_DEL_IN=false;
              ET_DEL_IN=0;
            state People_KID_IN
              en:
              WEIGHT=WEIGHT+30;
              KIDS=KIDS+1;
            state DELAY_IN
              state Set_tmr
                en:
                Q_DEL_IN=true;
              state Counting
                en:
                ET_DEL_IN = ET_DEL_IN + 1;
                Q_DEL_IN=false;
              state Set
                en:
                IN_DEL_IN=true;
                PT_DEL_IN=0.05;
              (junction 25127) -> Emergency.OpCl.OpCl_3.Opening3.People_IN.DELAY_IN.Set_tmr [order 1] : [ET_DEL_IN==PT_DEL_IN]
              Emergency.OpCl.OpCl_3.Opening3.People_IN.DELAY_IN.Set_tmr -> (junction 25128)
              Emergency.OpCl.OpCl_3.Opening3.People_IN.DELAY_IN.Counting -> (junction 25127)
              (junction 25127) -> (junction 25128) [order 2]
              (default) -> Emergency.OpCl.OpCl_3.Opening3.People_IN.DELAY_IN.Set
              Emergency.OpCl.OpCl_3.Opening3.People_IN.DELAY_IN.Set -> (junction 25129)
              (junction 25129) -> Emergency.OpCl.OpCl_3.Opening3.People_IN.DELAY_IN.Counting [order 1] : [ET_DEL_IN<PT_DEL_IN]
              (junction 25129) -> (junction 25128) [order 2]
            state People_WOMAN_IN
              en:
              WEIGHT=WEIGHT+55;
              WOMEN=WOMEN+1;
            state People_MAN_IN
              en:
              WEIGHT=WEIGHT+75;
              MEN=MEN+1;
            state People_FATGUY_IN
              en:
              WEIGHT=WEIGHT+100;
              FATGUYS=FATGUYS+1;
            state Re_Ready_IN
              en:
              COUNTER_IN=true;
            Emergency.OpCl.OpCl_3.Opening3.People_IN.Check_People_IN -> (junction 25072)
            (junction 25072) -> Emergency.OpCl.OpCl_3.Opening3.People_IN.People_KID_IN [order 1] : [KID_IN]
            Emergency.OpCl.OpCl_3.Opening3.People_IN.People_KID_IN -> (junction 25073)
            Emergency.OpCl.OpCl_3.Opening3.People_IN.DELAY_IN -> (junction 25074)
            (junction 25074) -> Emergency.OpCl.OpCl_3.Opening3.People_IN.Ready_IN [order 1] : [Q_DEL_IN]
            (default) -> Emergency.OpCl.OpCl_3.Opening3.People_IN.DELAY_IN
            Emergency.OpCl.OpCl_3.Opening3.People_IN.Ready_IN -> (junction 25075)
            (junction 25075) -> Emergency.OpCl.OpCl_3.Opening3.People_IN.Check_People_IN [order 1] : [COUNTER_IN]
            (junction 25072) -> (junction 25077) [order 2]
            (junction 25073) -> (junction 25076)
            (junction 25074) -> (junction 25086) [order 2]
            (junction 25075) -> (junction 25085) [order 2]
            (junction 25077) -> Emergency.OpCl.OpCl_3.Opening3.People_IN.People_WOMAN_IN [order 1] : [WOMAN_IN]
            Emergency.OpCl.OpCl_3.Opening3.People_IN.People_WOMAN_IN -> (junction 25076)
            (junction 25077) -> (junction 25078) [order 2]
            (junction 25076) -> (junction 25079)
            (junction 25078) -> Emergency.OpCl.OpCl_3.Opening3.People_IN.People_MAN_IN [order 1] : [MAN_IN]
            Emergency.OpCl.OpCl_3.Opening3.People_IN.People_MAN_IN -> (junction 25079)
            (junction 25078) -> (junction 25080) [order 2]
            (junction 25079) -> (junction 25081)
            (junction 25080) -> Emergency.OpCl.OpCl_3.Opening3.People_IN.People_FATGUY_IN [order 1] : [FATGUY_IN]
            Emergency.OpCl.OpCl_3.Opening3.People_IN.People_FATGUY_IN -> (junction 25081)
            (junction 25080) -> (junction 25082) [order 2]
            (junction 25081) -> (junction 25083)
            (junction 25082) -> (junction 25083)
            (junction 25083) -> (junction 25084)
            (junction 25085) -> (junction 25084)
            (junction 25084) -> (junction 25087)
            (junction 25086) -> (junction 25087)
            (junction 25087) -> (junction 25088)
            (junction 25088) -> Emergency.OpCl.OpCl_3.Opening3.People_IN.Re_Ready_IN [order 1] : [not(KID_IN|| WOMAN_IN || MAN_IN || FATGUY_IN)]
            (junction 25088) -> (junction 25089) [order 2]
            Emergency.OpCl.OpCl_3.Opening3.People_IN.Re_Ready_IN -> (junction 25089)
          state People_OUT
            state Ready_OUT
              en:
              IN_DEL_OUT=false;
              ET_DEL_OUT=0;
            state Check_People_OUT
              en:
              COUNTER_OUT=false;
            state People_KID_OUT
              en:
              WEIGHT=WEIGHT-30;
              KIDS=KIDS-1;
            state DELAY_OUT
              state Set_tmr
                en:
                Q_DEL_OUT=true;
              state Counting
                en:
                ET_DEL_OUT = ET_DEL_OUT + 1;
                Q_DEL_OUT=false;
              state Set
                en:
                IN_DEL_OUT=true;
                PT_DEL_OUT=0.05;
              (junction 25201) -> Emergency.OpCl.OpCl_3.Opening3.People_OUT.DELAY_OUT.Set_tmr [order 1] : [ET_DEL_OUT==PT_DEL_OUT]
              Emergency.OpCl.OpCl_3.Opening3.People_OUT.DELAY_OUT.Set_tmr -> (junction 25202)
              Emergency.OpCl.OpCl_3.Opening3.People_OUT.DELAY_OUT.Counting -> (junction 25201)
              (junction 25201) -> (junction 25202) [order 2]
              (default) -> Emergency.OpCl.OpCl_3.Opening3.People_OUT.DELAY_OUT.Set
              Emergency.OpCl.OpCl_3.Opening3.People_OUT.DELAY_OUT.Set -> (junction 25203)
              (junction 25203) -> Emergency.OpCl.OpCl_3.Opening3.People_OUT.DELAY_OUT.Counting [order 1] : [ET_DEL_OUT<PT_DEL_OUT]
              (junction 25203) -> (junction 25202) [order 2]
            state People_WOMAN_OUT
              en:
              WEIGHT=WEIGHT-55;
              WOMEN=WOMEN-1;
            state People_MAN_OUT
              en:
              WEIGHT=WEIGHT-75;
              MEN=MEN-1;
            state People_FATGUY_OUT
              en:
              WEIGHT=WEIGHT-100;
              FATGUYS=FATGUYS-1;
            state Re_Ready_OUT
              en:
              COUNTER_OUT=true;
            (default) -> Emergency.OpCl.OpCl_3.Opening3.People_OUT.DELAY_OUT
            Emergency.OpCl.OpCl_3.Opening3.People_OUT.DELAY_OUT -> (junction 25146)
            (junction 25146) -> Emergency.OpCl.OpCl_3.Opening3.People_OUT.Ready_OUT [order 1] : [Q_DEL_OUT]
            Emergency.OpCl.OpCl_3.Opening3.People_OUT.Ready_OUT -> (junction 25147)
            (junction 25147) -> Emergency.OpCl.OpCl_3.Opening3.People_OUT.Check_People_OUT [order 1] : [COUNTER_OUT]
            Emergency.OpCl.OpCl_3.Opening3.People_OUT.Check_People_OUT -> (junction 25148)
            (junction 25148) -> Emergency.OpCl.OpCl_3.Opening3.People_OUT.People_KID_OUT [order 1] : [KID_OUT && KIDS>0 ]
            Emergency.OpCl.OpCl_3.Opening3.People_OUT.People_KID_OUT -> (junction 25149)
            (junction 25146) -> (junction 25160) [order 2]
            (junction 25147) -> (junction 25158) [order 2]
            (junction 25148) -> (junction 25150) [order 2]
            (junction 25149) -> (junction 25151)
            (junction 25150) -> Emergency.OpCl.OpCl_3.Opening3.People_OUT.People_WOMAN_OUT [order 1] : [WOMAN_OUT && WOMEN>0]
            Emergency.OpCl.OpCl_3.Opening3.People_OUT.People_WOMAN_OUT -> (junction 25151)
            (junction 25150) -> (junction 25153) [order 2]
            (junction 25151) -> (junction 25152)
            (junction 25153) -> Emergency.OpCl.OpCl_3.Opening3.People_OUT.People_MAN_OUT [order 1] : [MAN_OUT && MEN>0]
            Emergency.OpCl.OpCl_3.Opening3.People_OUT.People_MAN_OUT -> (junction 25152)
            (junction 25153) -> (junction 25154) [order 2]
            (junction 25152) -> (junction 25155)
            (junction 25154) -> Emergency.OpCl.OpCl_3.Opening3.People_OUT.People_FATGUY_OUT [order 1] : [FATGUY_OUT && FATGUYS>0]
            Emergency.OpCl.OpCl_3.Opening3.People_OUT.People_FATGUY_OUT -> (junction 25155)
            (junction 25154) -> (junction 25157) [order 2]
            (junction 25155) -> (junction 25156)
            (junction 25157) -> (junction 25156)
            (junction 25156) -> (junction 25159)
            (junction 25158) -> (junction 25159)
            (junction 25159) -> (junction 25161)
            (junction 25160) -> (junction 25161)
            (junction 25161) -> (junction 25162)
            (junction 25162) -> Emergency.OpCl.OpCl_3.Opening3.People_OUT.Re_Ready_OUT [order 1] : [not(KID_OUT || WOMAN_OUT || MAN_OUT || FATGUY_OUT)]
            (junction 25162) -> (junction 25163) [order 2]
            Emergency.OpCl.OpCl_3.Opening3.People_OUT.Re_Ready_OUT -> (junction 25163)
          state Stop_Opening1
            en: AP3=false;
            FLAG_OD=true;
            IN_cl=false;
            ET_cl=0;
          Emergency.OpCl.OpCl_3.Opening3.Opening -> (junction 24942)
          (junction 24942) -> (junction 24941)
          Emergency.OpCl.OpCl_3.Opening3.Stop_Opening -> (junction 24942)
          (junction 24941) -> (junction 24945)
          (junction 24944) -> Emergency.OpCl.OpCl_3.Opening3.Opening [order 1] : [not(PA3)]
          Emergency.OpCl.OpCl_3.Opening3.BUTT_Temp -> (junction 24944)
          (junction 24944) -> Emergency.OpCl.OpCl_3.Opening3.Stop_Opening [order 2]
          Emergency.OpCl.OpCl_3.Opening3.Timer_open -> (junction 24943)
          (junction 24943) -> Emergency.OpCl.OpCl_3.Opening3.BUTT_Temp [order 1] : [not(FLAG==4)]
          (junction 24943) -> (junction 24944) [order 2]
          (junction 24947) -> Emergency.OpCl.OpCl_3.Opening3.Timer_open [order 1] : [not(OBS)]
          Emergency.OpCl.OpCl_3.Opening3.Opening1 -> (junction 24945)
          Emergency.OpCl.OpCl_3.Opening3.BUTT_Temp1 -> (junction 24946)
          (junction 24946) -> Emergency.OpCl.OpCl_3.Opening3.Opening1 [order 1] : [not(PA3)]
          Emergency.OpCl.OpCl_3.Opening3.People_IN -> Emergency.OpCl.OpCl_3.Opening3.People_OUT
          Emergency.OpCl.OpCl_3.Opening3.People_OUT -> (junction 24947)
          (junction 24947) -> (junction 24948) [order 2]
          (junction 24948) -> Emergency.OpCl.OpCl_3.Opening3.BUTT_Temp1 [order 1] : [not(FLAG==4)]
          (default) -> Emergency.OpCl.OpCl_3.Opening3.People_IN
          (junction 24948) -> (junction 24946) [order 2]
          (junction 24949) -> (junction 24945)
          (junction 24946) -> Emergency.OpCl.OpCl_3.Opening3.Stop_Opening1 [order 2]
          Emergency.OpCl.OpCl_3.Opening3.Stop_Opening1 -> (junction 24949)
        (default) -> (junction 24834)
        (junction 24834) -> (junction 24835) [order 1] : [FLAG_OD]
        (junction 24835) -> Emergency.OpCl.OpCl_3.Closing3 [order 1] : [not(SWITCH) && not(STOP) && WEIGHT<=320 && not(PD3 || P3) ]
        (junction 24834) -> Emergency.OpCl.OpCl_3.Opening3 [order 2]
        (junction 24835) -> Emergency.OpCl.OpCl_3.StopClosing [order 2]
        Emergency.OpCl.OpCl_3.Closing3 -> (junction 24836)
        Emergency.OpCl.OpCl_3.StopClosing -> (junction 24836)
        (junction 24836) -> (junction 24837)
        Emergency.OpCl.OpCl_3.Opening3 -> (junction 24837)
      state Closing0
        state BUTT_Temp
          state Butt_temp0
            en: BUT_TEMP = 0;
            FLAG_BT=true;
            LPC0=true;
          state Butt_temp1
            en: BUT_TEMP = 1;
            FLAG_BT=true;
            LPC1=true;
          state Butt_temp2
            en: BUT_TEMP = 2;
            FLAG_BT=true;
            LPC2=true;
          state Butt_temp3
            en: BUT_TEMP = 3;
            FLAG_BT=true;
            LPC3=true;
          (default) -> (junction 18130)
          (junction 18130) -> (junction 18131) [order 1] : [not(FLAG_BT)]
          (junction 18131) -> Emergency.OpCl.Closing0.BUTT_Temp.Butt_temp0 [order 1] : [P0]
          Emergency.OpCl.Closing0.BUTT_Temp.Butt_temp0 -> (junction 18132)
          (junction 18130) -> (junction 18139) [order 2]
          (junction 18131) -> (junction 18134) [order 2]
          (junction 18132) -> (junction 18133)
          (junction 18134) -> Emergency.OpCl.Closing0.BUTT_Temp.Butt_temp1 [order 1] : [P1]
          Emergency.OpCl.Closing0.BUTT_Temp.Butt_temp1 -> (junction 18133)
          (junction 18134) -> (junction 18135) [order 2]
          (junction 18133) -> (junction 18136)
          (junction 18135) -> Emergency.OpCl.Closing0.BUTT_Temp.Butt_temp2 [order 1] : [P2]
          Emergency.OpCl.Closing0.BUTT_Temp.Butt_temp2 -> (junction 18136)
          (junction 18135) -> (junction 18137) [order 2]
          (junction 18136) -> (junction 18138)
          (junction 18137) -> Emergency.OpCl.Closing0.BUTT_Temp.Butt_temp3 [order 1] : [P3]
          Emergency.OpCl.Closing0.BUTT_Temp.Butt_temp3 -> (junction 18138)
          (junction 18137) -> (junction 18140) [order 2]
          (junction 18138) -> (junction 18141)
          (junction 18139) -> (junction 18140)
          (junction 18140) -> (junction 18141)
        state Timer_close
          state Set_tmr
            en: Q_cl=true;
          state Set
            en:PT_cl=5;
            IN_cl=true;
          state Counting
            en:ET_cl = ET_cl + 1;
            Q_cl=false;
          (junction 18115) -> Emergency.OpCl.Closing0.Timer_close.Set_tmr [order 1] : [ET_cl==PT_cl]
          Emergency.OpCl.Closing0.Timer_close.Set_tmr -> (junction 18116)
          (default) -> Emergency.OpCl.Closing0.Timer_close.Set
          Emergency.OpCl.Closing0.Timer_close.Counting -> (junction 18115)
          (junction 18115) -> (junction 18116) [order 2]
          Emergency.OpCl.Closing0.Timer_close.Set -> (junction 18117)
          (junction 18117) -> Emergency.OpCl.Closing0.Timer_close.Counting [order 1] : [ET_cl<PT_cl]
          (junction 18117) -> (junction 18116) [order 2]
        state Closing
          en: CP0=Q_cl;
        state Stop_Closing
          en: CP0=false;
          LPS0=false;
          LPS1=false;
          LPD1=false;
          LPS2=false;
          LPD2=false;
          LPD3=false;
          FLAG_OD=false;
          OBS=false;
          ET_cl=0;
          IN_cl=false;
        state Flag_position
          en:FLAG=2;
          FLAG_BT=false;
          BUTTON=BUT_TEMP;
        state Closing1
          en:CP0=true;
        state Flag_floor
          en: FLAG=1;
        state Stop_Closing1
          en:CP0=false;
        Emergency.OpCl.Closing0.Closing -> Emergency.OpCl.Closing0.BUTT_Temp
        (default) -> (junction 18082)
        (junction 18082) -> Emergency.OpCl.Closing0.Timer_close [order 1] : [not(FLAG==0) && not(FLAG==4)]
        Emergency.OpCl.Closing0.Timer_close -> (junction 18083)
        (junction 18083) -> Emergency.OpCl.Closing0.Closing [order 1] : [not(PC0)]
        Emergency.OpCl.Closing0.BUTT_Temp -> (junction 18084)
        (junction 18082) -> (junction 18086) [order 2]
        (junction 18083) -> Emergency.OpCl.Closing0.Stop_Closing [order 2]
        (junction 18084) -> (junction 18088)
        Emergency.OpCl.Closing0.Stop_Closing -> (junction 18085)
        (junction 18085) -> Emergency.OpCl.Closing0.Flag_position [order 1] : [FLAG_BT]
        (junction 18085) -> Emergency.OpCl.Closing0.Flag_floor [order 2]
        Emergency.OpCl.Closing0.Flag_position -> (junction 18089)
        (junction 18086) -> Emergency.OpCl.Closing0.Closing1 [order 1] : [not(PC0)]
        Emergency.OpCl.Closing0.Closing1 -> (junction 18087)
        (junction 18086) -> Emergency.OpCl.Closing0.Stop_Closing1 [order 2]
        (junction 18087) -> (junction 18090)
        Emergency.OpCl.Closing0.Flag_floor -> (junction 18089)
        (junction 18089) -> (junction 18088)
        (junction 18088) -> (junction 18091)
        Emergency.OpCl.Closing0.Stop_Closing1 -> (junction 18090)
        (junction 18090) -> (junction 18091)
      state Closing1
        state Timer_close
          state Set_tmr
            en: Q_cl=true;
          state Set
            en:PT_cl=5;
            IN_cl=true;
          state Counting
            en:ET_cl = ET_cl + 1;
            Q_cl=false;
          (junction 18397) -> Emergency.OpCl.Closing1.Timer_close.Set_tmr [order 1] : [ET_cl==PT_cl]
          Emergency.OpCl.Closing1.Timer_close.Set_tmr -> (junction 18398)
          (default) -> Emergency.OpCl.Closing1.Timer_close.Set
          Emergency.OpCl.Closing1.Timer_close.Counting -> (junction 18397)
          (junction 18397) -> (junction 18398) [order 2]
          Emergency.OpCl.Closing1.Timer_close.Set -> (junction 18399)
          (junction 18399) -> Emergency.OpCl.Closing1.Timer_close.Counting [order 1] : [ET_cl<PT_cl]
          (junction 18399) -> (junction 18398) [order 2]
        state BUTT_Temp
          state Butt_temp0
            en: BUT_TEMP = 0;
            FLAG_BT=true;
            LPC0=true;
          state Butt_temp1
            en: BUT_TEMP = 1;
            FLAG_BT=true;
            LPC1=true;
          state Butt_temp2
            en: BUT_TEMP = 2;
            FLAG_BT=true;
            LPC2=true;
          state Butt_temp3
            en: BUT_TEMP = 3;
            FLAG_BT=true;
            LPC3=true;
          (default) -> (junction 18412)
          (junction 18412) -> (junction 18413) [order 1] : [not(FLAG_BT)]
          (junction 18413) -> Emergency.OpCl.Closing1.BUTT_Temp.Butt_temp0 [order 1] : [P0]
          Emergency.OpCl.Closing1.BUTT_Temp.Butt_temp0 -> (junction 18414)
          (junction 18412) -> (junction 18421) [order 2]
          (junction 18413) -> (junction 18416) [order 2]
          (junction 18414) -> (junction 18415)
          (junction 18416) -> Emergency.OpCl.Closing1.BUTT_Temp.Butt_temp1 [order 1] : [P1]
          Emergency.OpCl.Closing1.BUTT_Temp.Butt_temp1 -> (junction 18415)
          (junction 18416) -> (junction 18417) [order 2]
          (junction 18415) -> (junction 18418)
          (junction 18417) -> Emergency.OpCl.Closing1.BUTT_Temp.Butt_temp2 [order 1] : [P2]
          Emergency.OpCl.Closing1.BUTT_Temp.Butt_temp2 -> (junction 18418)
          (junction 18417) -> (junction 18419) [order 2]
          (junction 18418) -> (junction 18420)
          (junction 18419) -> Emergency.OpCl.Closing1.BUTT_Temp.Butt_temp3 [order 1] : [P3]
          Emergency.OpCl.Closing1.BUTT_Temp.Butt_temp3 -> (junction 18420)
          (junction 18419) -> (junction 18422) [order 2]
          (junction 18420) -> (junction 18423)
          (junction 18421) -> (junction 18422)
          (junction 18422) -> (junction 18423)
        state Closing
          en: CP1=Q_cl;
        state Stop_Closing
          en: CP1=false;
          LPS0=false;
          LPS1=false;
          LPD1=false;
          LPS2=false;
          LPD2=false;
          LPD3=false;
          FLAG_OD=false;
          OBS=false;
          ET_cl=0;
          IN_cl=false;
        state Flag_position
          en:FLAG=2;
          FLAG_BT=false;
          BUTTON=BUT_TEMP;
        state Closing1
          en:CP1=true;
        state Flag_floor
          en: FLAG=1;
        state Stop_Closing1
          en:CP1=false;
        Emergency.OpCl.Closing1.Closing -> Emergency.OpCl.Closing1.BUTT_Temp
        (default) -> (junction 18364)
        (junction 18364) -> Emergency.OpCl.Closing1.Timer_close [order 1] : [not(FLAG==0) && not(FLAG==4)]
        Emergency.OpCl.Closing1.Timer_close -> (junction 18365)
        Emergency.OpCl.Closing1.BUTT_Temp -> (junction 18366)
        (junction 18365) -> Emergency.OpCl.Closing1.Closing [order 1] : [not(PC1)]
        (junction 18364) -> (junction 18368) [order 2]
        (junction 18365) -> Emergency.OpCl.Closing1.Stop_Closing [order 2]
        (junction 18366) -> (junction 18370)
        Emergency.OpCl.Closing1.Stop_Closing -> (junction 18367)
        (junction 18367) -> Emergency.OpCl.Closing1.Flag_position [order 1] : [FLAG_BT]
        (junction 18367) -> Emergency.OpCl.Closing1.Flag_floor [order 2]
        Emergency.OpCl.Closing1.Flag_position -> (junction 18371)
        (junction 18368) -> Emergency.OpCl.Closing1.Closing1 [order 1] : [not(PC1)]
        Emergency.OpCl.Closing1.Closing1 -> (junction 18369)
        (junction 18368) -> Emergency.OpCl.Closing1.Stop_Closing1 [order 2]
        (junction 18369) -> (junction 18372)
        Emergency.OpCl.Closing1.Flag_floor -> (junction 18371)
        (junction 18371) -> (junction 18370)
        (junction 18370) -> (junction 18373)
        Emergency.OpCl.Closing1.Stop_Closing1 -> (junction 18372)
        (junction 18372) -> (junction 18373)
      state Closing2
        state BUTT_Temp
          state Butt_temp0
            en: BUT_TEMP = 0;
            FLAG_BT=true;
            LPC0=true;
          state Butt_temp1
            en: BUT_TEMP = 1;
            FLAG_BT=true;
            LPC1=true;
          state Butt_temp2
            en: BUT_TEMP = 2;
            FLAG_BT=true;
            LPC2=true;
          state Butt_temp3
            en: BUT_TEMP = 3;
            FLAG_BT=true;
            LPC3=true;
          (default) -> (junction 18504)
          (junction 18504) -> (junction 18505) [order 1] : [not(FLAG_BT)]
          (junction 18505) -> Emergency.OpCl.Closing2.BUTT_Temp.Butt_temp0 [order 1] : [P0]
          Emergency.OpCl.Closing2.BUTT_Temp.Butt_temp0 -> (junction 18506)
          (junction 18504) -> (junction 18513) [order 2]
          (junction 18505) -> (junction 18508) [order 2]
          (junction 18506) -> (junction 18507)
          (junction 18508) -> Emergency.OpCl.Closing2.BUTT_Temp.Butt_temp1 [order 1] : [P1]
          Emergency.OpCl.Closing2.BUTT_Temp.Butt_temp1 -> (junction 18507)
          (junction 18508) -> (junction 18509) [order 2]
          (junction 18507) -> (junction 18510)
          (junction 18509) -> Emergency.OpCl.Closing2.BUTT_Temp.Butt_temp2 [order 1] : [P2]
          Emergency.OpCl.Closing2.BUTT_Temp.Butt_temp2 -> (junction 18510)
          (junction 18509) -> (junction 18511) [order 2]
          (junction 18510) -> (junction 18512)
          (junction 18511) -> Emergency.OpCl.Closing2.BUTT_Temp.Butt_temp3 [order 1] : [P3]
          Emergency.OpCl.Closing2.BUTT_Temp.Butt_temp3 -> (junction 18512)
          (junction 18511) -> (junction 18514) [order 2]
          (junction 18512) -> (junction 18515)
          (junction 18513) -> (junction 18514)
          (junction 18514) -> (junction 18515)
        state Timer_close
          state Set_tmr
            en: Q_cl=true;
          state Set
            en:PT_cl=5;
            IN_cl=true;
          state Counting
            en:ET_cl = ET_cl + 1;
            Q_cl=false;
          (junction 18489) -> Emergency.OpCl.Closing2.Timer_close.Set_tmr [order 1] : [ET_cl==PT_cl]
          Emergency.OpCl.Closing2.Timer_close.Set_tmr -> (junction 18490)
          (default) -> Emergency.OpCl.Closing2.Timer_close.Set
          Emergency.OpCl.Closing2.Timer_close.Counting -> (junction 18489)
          (junction 18489) -> (junction 18490) [order 2]
          Emergency.OpCl.Closing2.Timer_close.Set -> (junction 18491)
          (junction 18491) -> Emergency.OpCl.Closing2.Timer_close.Counting [order 1] : [ET_cl<PT_cl]
          (junction 18491) -> (junction 18490) [order 2]
        state Closing
          en: CP2=Q_cl;
        state Stop_Closing
          en: CP2=false;
          LPS0=false;
          LPS1=false;
          LPD1=false;
          LPS2=false;
          LPD2=false;
          LPD3=false;
          FLAG_OD=false;
          OBS=false;
          ET_cl=0;
          IN_cl=false;
        state Flag_position
          en:FLAG=2;
          FLAG_BT=false;
          BUTTON=BUT_TEMP;
        state Closing1
          en:CP2=true;
        state Flag_floor
          en: FLAG=1;
        state Stop_Closing1
          en:CP2=false;
        Emergency.OpCl.Closing2.Closing -> Emergency.OpCl.Closing2.BUTT_Temp
        (default) -> (junction 18456)
        (junction 18456) -> Emergency.OpCl.Closing2.Timer_close [order 1] : [not(FLAG==0) && not(FLAG==4)]
        Emergency.OpCl.Closing2.Timer_close -> (junction 18457)
        (junction 18457) -> Emergency.OpCl.Closing2.Closing [order 1] : [not(PC2)]
        Emergency.OpCl.Closing2.BUTT_Temp -> (junction 18458)
        (junction 18456) -> (junction 18460) [order 2]
        (junction 18457) -> Emergency.OpCl.Closing2.Stop_Closing [order 2]
        (junction 18458) -> (junction 18462)
        Emergency.OpCl.Closing2.Stop_Closing -> (junction 18459)
        (junction 18459) -> Emergency.OpCl.Closing2.Flag_position [order 1] : [FLAG_BT]
        (junction 18459) -> Emergency.OpCl.Closing2.Flag_floor [order 2]
        Emergency.OpCl.Closing2.Flag_position -> (junction 18463)
        (junction 18460) -> Emergency.OpCl.Closing2.Closing1 [order 1] : [not(PC2)]
        Emergency.OpCl.Closing2.Closing1 -> (junction 18461)
        (junction 18460) -> Emergency.OpCl.Closing2.Stop_Closing1 [order 2]
        (junction 18461) -> (junction 18464)
        Emergency.OpCl.Closing2.Flag_floor -> (junction 18463)
        (junction 18463) -> (junction 18462)
        (junction 18462) -> (junction 18465)
        Emergency.OpCl.Closing2.Stop_Closing1 -> (junction 18464)
        (junction 18464) -> (junction 18465)
      state Closing3
        state BUTT_Temp
          state Butt_temp0
            en: BUT_TEMP = 0;
            FLAG_BT=true;
            LPC0=true;
          state Butt_temp1
            en: BUT_TEMP = 1;
            FLAG_BT=true;
            LPC1=true;
          state Butt_temp2
            en: BUT_TEMP = 2;
            FLAG_BT=true;
            LPC2=true;
          state Butt_temp3
            en: BUT_TEMP = 3;
            FLAG_BT=true;
            LPC3=true;
          (default) -> (junction 18596)
          (junction 18596) -> (junction 18597) [order 1] : [not(FLAG_BT)]
          (junction 18597) -> Emergency.OpCl.Closing3.BUTT_Temp.Butt_temp0 [order 1] : [P0]
          Emergency.OpCl.Closing3.BUTT_Temp.Butt_temp0 -> (junction 18598)
          (junction 18596) -> (junction 18605) [order 2]
          (junction 18597) -> (junction 18600) [order 2]
          (junction 18598) -> (junction 18599)
          (junction 18600) -> Emergency.OpCl.Closing3.BUTT_Temp.Butt_temp1 [order 1] : [P1]
          Emergency.OpCl.Closing3.BUTT_Temp.Butt_temp1 -> (junction 18599)
          (junction 18600) -> (junction 18601) [order 2]
          (junction 18599) -> (junction 18602)
          (junction 18601) -> Emergency.OpCl.Closing3.BUTT_Temp.Butt_temp2 [order 1] : [P2]
          Emergency.OpCl.Closing3.BUTT_Temp.Butt_temp2 -> (junction 18602)
          (junction 18601) -> (junction 18603) [order 2]
          (junction 18602) -> (junction 18604)
          (junction 18603) -> Emergency.OpCl.Closing3.BUTT_Temp.Butt_temp3 [order 1] : [P3]
          Emergency.OpCl.Closing3.BUTT_Temp.Butt_temp3 -> (junction 18604)
          (junction 18603) -> (junction 18606) [order 2]
          (junction 18604) -> (junction 18607)
          (junction 18605) -> (junction 18606)
          (junction 18606) -> (junction 18607)
        state Timer_close
          state Set_tmr
            en: Q_cl=true;
          state Set
            en:PT_cl=5;
            IN_cl=true;
          state Counting
            en:ET_cl = ET_cl + 1;
            Q_cl=false;
          (junction 18581) -> Emergency.OpCl.Closing3.Timer_close.Set_tmr [order 1] : [ET_cl==PT_cl]
          Emergency.OpCl.Closing3.Timer_close.Set_tmr -> (junction 18582)
          (default) -> Emergency.OpCl.Closing3.Timer_close.Set
          Emergency.OpCl.Closing3.Timer_close.Counting -> (junction 18581)
          (junction 18581) -> (junction 18582) [order 2]
          Emergency.OpCl.Closing3.Timer_close.Set -> (junction 18583)
          (junction 18583) -> Emergency.OpCl.Closing3.Timer_close.Counting [order 1] : [ET_cl<PT_cl]
          (junction 18583) -> (junction 18582) [order 2]
        state Closing
          en: CP3=Q_cl;
        state Stop_Closing
          en: CP3=false;
          LPS0=false;
          LPS1=false;
          LPD1=false;
          LPS2=false;
          LPD2=false;
          LPD3=false;
          FLAG_OD=false;
          OBS=false;
          ET_cl=0;
          IN_cl=false;
        state Flag_position
          en:FLAG=2;
          FLAG_BT=false;
          BUTTON=BUT_TEMP;
        state Closing1
          en:CP3=true;
        state Flag_floor
          en: FLAG=1;
        state Stop_Closing1
          en:CP3=false;
        Emergency.OpCl.Closing3.Closing -> Emergency.OpCl.Closing3.BUTT_Temp
        (default) -> (junction 18548)
        (junction 18548) -> Emergency.OpCl.Closing3.Timer_close [order 1] : [not(FLAG==0) && not(FLAG==4)]
        Emergency.OpCl.Closing3.Timer_close -> (junction 18549)
        (junction 18549) -> Emergency.OpCl.Closing3.Closing [order 1] : [not(PC3)]
        Emergency.OpCl.Closing3.BUTT_Temp -> (junction 18550)
        (junction 18548) -> (junction 18552) [order 2]
        (junction 18549) -> Emergency.OpCl.Closing3.Stop_Closing [order 2]
        (junction 18550) -> (junction 18554)
        Emergency.OpCl.Closing3.Stop_Closing -> (junction 18551)
        (junction 18551) -> Emergency.OpCl.Closing3.Flag_position [order 1] : [FLAG_BT]
        (junction 18551) -> Emergency.OpCl.Closing3.Flag_floor [order 2]
        Emergency.OpCl.Closing3.Flag_position -> (junction 18555)
        (junction 18552) -> Emergency.OpCl.Closing3.Closing1 [order 1] : [not(PC3)]
        Emergency.OpCl.Closing3.Closing1 -> (junction 18553)
        (junction 18552) -> Emergency.OpCl.Closing3.Stop_Closing1 [order 2]
        (junction 18553) -> (junction 18556)
        Emergency.OpCl.Closing3.Flag_floor -> (junction 18555)
        (junction 18555) -> (junction 18554)
        (junction 18554) -> (junction 18557)
        Emergency.OpCl.Closing3.Stop_Closing1 -> (junction 18556)
        (junction 18556) -> (junction 18557)
      FLOOR_0 -> Emergency.OpCl.OpCl_0
      (junction 4681) -> (junction 4675) [order 1] : [(SWITCH || FLAG_EMG || FLAG_BO) && (RPC0 || RPC1 || RPC2 || RPC3)]
      (junction 4675) -> FLOOR_0 [order 1] : [FLOOR==0]
      Emergency.OpCl.OpCl_0 -> (junction 16534)
      (default) -> (junction 4681)
      (junction 4681) -> (junction 4682) [order 2] : [not(BO) && FLAG_OD && not(FLAG_EMG)]
      (junction 16534) -> (junction 16535)
      (junction 4675) -> (junction 16528) [order 2]
      (junction 16528) -> FLOOR_1 [order 1] : [FLOOR==1]
      Emergency.OpCl.OpCl_1 -> (junction 16535)
      FLOOR_1 -> Emergency.OpCl.OpCl_1
      (junction 16528) -> (junction 16530) [order 2]
      (junction 16535) -> (junction 16536)
      (junction 16530) -> FLOOR_2 [order 1] : [FLOOR==2]
      Emergency.OpCl.OpCl_2 -> (junction 16536)
      FLOOR_2 -> Emergency.OpCl.OpCl_2
      (junction 16536) -> (junction 16537)
      (junction 16530) -> (junction 16532) [order 2]
      FLOOR_3 -> Emergency.OpCl.OpCl_3
      (junction 16532) -> FLOOR_3 [order 1] : [FLOOR==3]
      Emergency.OpCl.OpCl_3 -> (junction 16537)
      (junction 16532) -> (junction 16545) [order 2]
      (junction 16537) -> (junction 16545)
      (junction 16545) -> (junction 19537)
      (junction 4682) -> Emergency.OpCl.Closing0 [order 1] : [FLOOR==0]
      Emergency.OpCl.Closing0 -> (junction 18639)
      (junction 18639) -> (junction 18641)
      (junction 4682) -> (junction 18173) [order 2]
      (junction 18173) -> Emergency.OpCl.Closing1 [order 1] : [FLOOR==1]
      Emergency.OpCl.Closing1 -> (junction 18641)
      (junction 18641) -> (junction 18642)
      (junction 18173) -> (junction 18175) [order 2]
      (junction 18175) -> Emergency.OpCl.Closing2 [order 1] : [FLOOR==2]
      Emergency.OpCl.Closing2 -> (junction 18642)
      (junction 18175) -> (junction 18176) [order 2]
      (junction 18642) -> (junction 18643)
      (junction 18176) -> Emergency.OpCl.Closing3 [order 1] : [FLOOR==3]
      Emergency.OpCl.Closing3 -> (junction 18643)
      (junction 18176) -> (junction 19534) [order 2]
      (junction 18643) -> (junction 19534)
      (junction 19534) -> (junction 19537)
    state Replaced
      en:
      SCENDI=false;
    state NOT_EME
      en:
      FLAG_EMG=false;
    state Timer_EME_OFF
      state Set_tmr
        en: Q_EME_OFF=true;
      state Counting
        en:ET_EME_OFF = ET_EME_OFF + 1;
        Q_EME_OFF=false;
      state Set
        en:PT_EME_OFF=3;
        IN_EME_OFF=true;
      (junction 13253) -> Emergency.Timer_EME_OFF.Set_tmr [order 1] : [ET_EME_OFF==PT_EME_OFF]
      Emergency.Timer_EME_OFF.Set_tmr -> (junction 13254)
      Emergency.Timer_EME_OFF.Counting -> (junction 13253)
      (junction 13253) -> (junction 13254) [order 2]
      (default) -> Emergency.Timer_EME_OFF.Set
      Emergency.Timer_EME_OFF.Set -> (junction 13255)
      (junction 13255) -> Emergency.Timer_EME_OFF.Counting [order 1] : [ET_EME_OFF<PT_EME_OFF]
      (junction 13255) -> (junction 13254) [order 2]
    state KEEP_EME
      en:
      IN_EME_OFF=false;
      ET_EME_OFF=0;
    state NOT_BO
      en:
      FLAG_BO=false;
    state EME_FINISH
      en: FLAG=1;
      LPS0=false; LPS1=false;
      LPD1=false; LPS2=false;
      LPD2=false; LPD3=false;
      OBS=false; FLAG_OD=false;
      IN_cl=false; ET_cl=0;
      IN_EME=false; ET_EME=0;
      IN_EME_OFF=false; ET_EME_OFF=0;
      FIRST=true; FLAG_REC=false;
    FIRST -> (junction 4618)
    (junction 4618) -> Emergency.Replacing [order 1] : [not(RPC0) && not(RPC1) && not(RPC2) && not(RPC3)]
    (default) -> (junction 16475)
    (junction 16475) -> BLK_Eme [order 1] : [FLAG_EMG]
    BLK_Eme -> (junction 16477)
    (junction 16477) -> REC [order 1] : [FLAG_REC && BO]
    REC -> (junction 16479)
    (junction 16479) -> FIRST [order 1] : [FIRST]
    (junction 16479) -> (junction 4618) [order 2]
    (junction 16477) -> (junction 16479) [order 2]
    (junction 16475) -> (junction 16477) [order 2]
    (junction 4618) -> Emergency.Replaced [order 2]
    Emergency.Replacing -> (junction 16498)
    (junction 16498) -> OpCl
    Emergency.Replaced -> (junction 16498)
    OpCl -> (junction 16524)
    (junction 16524) -> (junction 16523)
    (junction 16523) -> (junction 16518)
    (junction 16518) -> (junction 13250) [order 1] : [((not(BO) && not(FLAG_REC)) || FLAG_EMG) && not(FIRE)]
    (junction 13250) -> Timer_EME_OFF [order 1] : [STOP && (PA0 || PA1|| PA2 || PA3)]
    Timer_EME_OFF -> (junction 16483)
    (junction 16483) -> NOT_EME [order 1] : [Q_EME_OFF]
    (junction 16518) -> (junction 16519) [order 2]
    (junction 13250) -> KEEP_EME [order 2]
    (junction 16483) -> (junction 16482) [order 2]
    NOT_EME -> (junction 16486)
    (junction 16482) -> (junction 16486)
    (junction 16486) -> (junction 16489)
    KEEP_EME -> (junction 16489)
    (junction 16489) -> (junction 16516)
    (junction 16519) -> (junction 16516)
    (junction 16516) -> (junction 25232)
    (junction 25232) -> (junction 16512) [order 2]
    (junction 25232) -> NOT_BO [order 1] : [(PA0 || PA1 || PA2 || PA3) && not(BO)]
    NOT_BO -> (junction 16512)
    (junction 16512) -> (junction 16493)
    (junction 16493) -> EME_FINISH [order 1] : [(RPC0 || RPC1 || RPC2 || RPC3) && (PC0 && PC1 && PC2 && PC3) && not(FLAG_EMG) && not(BO)]
    (junction 16493) -> (junction 16506) [order 2]
    EME_FINISH -> (junction 16508)
    (junction 16506) -> (junction 16508)
  Init_procedure -> (junction 13645)
  Floor_detection -> (junction 4471)
  (junction 4471) -> Init_procedure [order 1] : [FLAG==0]
  (default) -> Blackout
  Fire_detection -> Floor_detection
  Blackout -> Fire_detection
  (junction 13645) -> (junction 13646)
  (junction 4471) -> (junction 13586) [order 2]
  (junction 13658) -> Blackout
  (junction 13586) -> Button_detection [order 1] : [FLAG==1]
  Button_detection -> (junction 13646)
  (junction 13586) -> (junction 13588) [order 2]
  (junction 13646) -> (junction 13649)
  (junction 13588) -> Position_control [order 1] : [FLAG==2]
  Position_control -> (junction 13649)
  (junction 13588) -> (junction 13593) [order 2]
  (junction 13649) -> (junction 13648)
  (junction 13593) -> OpCl_doors [order 1] : [FLAG==3]
  OpCl_doors -> (junction 13648)
  (junction 13593) -> (junction 13596) [order 2]
  (junction 13648) -> (junction 4479)
  (junction 13596) -> Emergency [order 1] : [FLAG==4]
  Emergency -> (junction 4479)
  (junction 4479) -> (junction 13658)
  (junction 13596) -> (junction 13658) [order 2]
  data: FLAG local =0; STOP input boolean =false; BUTTON local =0; FLOOR local =0; SALI output =false; SCENDI output =false; PS1 input; PD1 input; P1 input; PD2 input; PS2 input; P2 input; PD3 input; P3 input; PS0 input; SWITCH input; P0 input; LPC3 output =false; LPC1 output =false; LPC0 output =false; LPC2 output =false; RPC2 input; RPC1 input; RPC3 input; RPC0 input; AP1 output =false; LPS0 output =false; LPS1 output =false; LPS2 output =false; CP3 output =false; LPD2 output =false; LPD1 output =false; LPD3 output =false; CP1 output =false; AP0 output =false; CP0 output =false; AP2 output =false; CP2 output =false; AP3 output =false; OBS local =false; FLAG_OD local =false; PC3 input; PC2 input; PC0 input; PC1 input; PA3 input; PA1 input; PA2 input; PA0 input; IN_LL local =false; IN_EME local =false; FLAG_EME local =false; IN_op local =false; IN_EME_OFF local =false; IN_cl local =false; IN_DEL_OUT local =false; IN_DEL_IN local =false; FIRST local =false; FLAG_BO local =false; Q_DEL_IN local =false; BUT_TEMP local =0; Q_op local =false; FLAG_BT local =false; PT_cl local =5; LL output =false; Q_LL local =false; ET_LL local =0; PT_LL local =10; Q_EME local =false; ET_EME local =0; PT_EME local =3; MOTION local =0; PT_op local =2; ET_EME_OFF local =0; FLAG_STOP local =false; Q_EME_OFF local =false; PT_EME_OFF local =3; ET_op local =0; WOMEN local =0; WEIGHT local =0; ET_cl local =0; FATGUYS local =0; Q_cl local =false; MEN local =0; KIDS local =0; Q_DEL_OUT local =false; COUNTER_IN local =false; ET_DEL_OUT local =0; ET_DEL_IN local =0; PT_DEL_IN local =0.05; PT_DEL_OUT local =0.05; COUNTER_OUT local =false; FLAG_REC local =false; FLAG_EMG local =false; RECOVERY local =false; MAN_OUT local =false; WOMAN_IN local =false; MAN_IN local =false; KID_IN local =false; KID_OUT local =false; WOMAN_OUT local =false; FATGUY_OUT local =false; FATGUY_IN local =false; BO input =false; FIRE input =false
